simulink model "Noh_Nofusion"  (R2020b)
settings: Solver=FixedStepAuto  StartTime=0.0  StopTime=Inf  FixedStep=0.01  RelTol=1e-3
PostLoadFcn:
  | if any(exist('dsrtsu_mdlpostloadfcn', 'file') ~= 0), dsrtsu_mdlpostloadfcn('Execute', bdroot); end
InitFcn:
  | , if any(exist('rtifpga_mdlclblib', 'file') ~= 0), rtifpga_mdlclblib('Init', bdroot); end,
  | , if any(exist('dsmpb_private', 'file') ~= 0), dsmpb_private('dsmpb_mdlclblib', 'Init', bdroot); end,
undefined symbols (not defined in the file): ACC_TimeGap_DecSetSwt, ACC_TimeGap_IncSetSwt, AccelPedalPosn, AccelPedalPosnVldty, AccelPedlPosnDiagc, AccPedalOverride, ACU_ShiftInProgress, ADAS_Posn_CurLane, AESSwtReq, ALC_SwtReq, BrkPedalSts, CC_ACC_CANCEL_OFFSwt, CC_ACC_CRUISE_OFFSwt, CC_ACC_DecSetSpd_SetSwt, CC_ACC_IncSetSpd_ResuSwt, CC_ACCSwtErr, CharSpd_ms, CSA_NODE, CURRENT_GEAR, CurrentGearValid, DiscIntNeverNeededParam, DrvDoorSts, DrvSBR, DrvTrqReqOvld, ECMACCInterface, ECMRespACC, ELKSwtReq, EngLimpHomeSts, EngSpd, EngState, EngState_PHEV, EngTrqMaxActSpd, EngTrqMinAct, EPS_DrvInpTrqVal_HighReslolution, EPS_FailSts, EPS_LKATorqOvrlDlvd, EPS_LKATorqOvrlDlvdVld, EPS_LKATrqOvlDlvdSts, EPS_SteerMod, EPS_TrqSnsrSts, EQ4_APPINFO, EQ4_LA_ELEM, EQ4_LA_HDR, EQ4_LAP_ELEM, EQ4_LAP_HDR, EQ4_LH_ELEM, EQ4_LH_HDR, EQ4_LRE_ELEM, EQ4_LRE_HDR, ESS_PedSwtReq, ESS_VehSwtReq, FFogLmpSts_F_Pbox, FLWheelDriveDirection, FLWheelSpd, FrntWiprSwtSts, FrntWshrSwtSts, FRWheelDriveDirection, FRWheelSpd, HazardLmpSwtSts, HCU_AccelPedalPosn_Diag ... (+153)
libraries: simulink x132, dsmpblib x27
(part 14 of 14)

== matlab function Noh_Nofusion/TOS/Subsystem1/ACCOSM/HWA_Task100ms1/DycHistCalc ==
  data: TrajHistBufferBTrajEnd input boolean; ObjTrajNumber input uint8; ObjDycHist output single; TrajCurrentIndex input uint8; TrajHistBufferBValid input boolean; TrajHistBufferDxv input single; TrajHistBufferDyv input single; ObjValid input boolean; ObjqDycHist output single; dxC0 input; aP0 input; bP0 input; cP0 input; aP1 input; bP1 input; cP1 input
function [ObjDycHist,ObjqDycHist] = DycHistCalc(TrajHistBufferBTrajEnd,ObjTrajNumber,TrajCurrentIndex,...
    TrajHistBufferBValid,TrajHistBufferDxv,TrajHistBufferDyv,ObjValid,dxC0,aP0,bP0,cP0,aP1,bP1,cP1)

t_dxv = single(0);
t_dyv = single(0);
t_dxvK1 = single(0);
t_dyvK1 = single(0);
ObjDycHist = single(zeros(15,1));
ObjqDycHist = single(zeros(15,1));

for iObj=1:15
    t_TrajNumber = ObjTrajNumber(iObj);
    if t_TrajNumber<21
        t_End = false;
        t_Failed = false;
        t_TrajCurrentIndex = TrajCurrentIndex(t_TrajNumber);
        t_TrajEnd = TrajHistBufferBTrajEnd(t_TrajNumber,t_TrajCurrentIndex);
        if (ObjValid(iObj)==true)&&(t_TrajEnd==false)
            for k=1:24
                if t_End==false
                    if t_TrajCurrentIndex<k
                        t_Index = t_TrajCurrentIndex + uint8(25) - k;
                    else
                        t_Index = t_TrajCurrentIndex - k + uint8(1);
                    end
                    if t_Index==1
                        t_IndexK1 = uint8(24);
                    else
                        t_IndexK1 = t_Index - uint8(1);
                    end
                    t_ValidK1 = TrajHistBufferBValid(t_TrajNumber,t_IndexK1);
                    t_TrajEndK1 = TrajHistBufferBTrajEnd(t_TrajNumber,t_IndexK1);
                    t_dxv = TrajHistBufferDxv(t_TrajNumber,t_Index);
                    t_dxvK1 = TrajHistBufferDxv(t_TrajNumber,t_IndexK1);
                    t_dyv = TrajHistBufferDyv(t_TrajNumber,t_Index);
                    t_dyvK1 = TrajHistBufferDyv(t_TrajNumber,t_IndexK1);
                    
                    if (t_TrajEndK1==true)||(t_ValidK1==false)
                        t_End = true;
                        t_Failed = true;
                    end
                    if (t_dxv>=0)&&(t_dxvK1<=0)
                        t_End = true;
                    end
                end
            end
        end
        if (t_End==true)&&(t_Failed==false)
            if (t_dxv==t_dxvK1)
                t_dycHist = t_dyv;
            else
                t_dycHist = t_dyv - t_dxv*(t_dyvK1 - t_dyv)/(t_dxvK1 - t_dxv);
            end
            t_qDycHist = single(1);  
        else
            if (t_End==true)&&(t_Failed==true)&&(t_dxv>0)
                if t_dxv>(dxC0)
                    t_dycHist = t_dyv - (aP1*t_dxv*t_dxv + bP1*t_dxv + cP1); 
                else
                    t_dycHist = t_dyv - (aP0*t_dxv*t_dxv + bP0*t_dxv + cP0); 
                end
               t_qDycHist = max((single(80) - t_dxv)/single(80),single(0));
            else
                t_dycHist = single(0);
                t_qDycHist = single(0);
            end
        end
    else
        t_dycHist = single(0);
        t_qDycHist = single(0);
    end
    ObjDycHist(iObj) = t_dycHist;
    ObjqDycHist(iObj) = t_qDycHist;
end

== matlab function Noh_Nofusion/TOS/Subsystem1/ACCOSM/HWA_Task100ms1/LostTargetCalc ==
  data: ObjValid input boolean size=15; ReID output uint8 size=1; ObjDx input single size=15; ObjDy input single size=15; DeltaDx input single size=1; DeltaDy input single size=1; P0IDK1 input uint8 size=1; P0VxK1 input single size=1; P0DxK1 input single size=1; P0DyK1 input single size=1; P0RangeK1 input; P0ArGK1 input; P0DycK1 input single size=1; P0VycK1 input single size=1; P0CutIn_bK1 input boolean size=1; tTargetLostK1 input single size=1; ReRange output single size=1; ReArG output single size=1; ReDx output single size=1; ReDy output single size=1; ReVx output single size=1; ReCutIn_b output boolean size=1; ReDyc output single size=1; ReVyc output single size=1; TargetLost_b output boolean size=1; Covered_b output boolean size=1; tTargetLost output single size=1
function [ReID,ReRange,ReArG,ReDx,ReDy,ReVx,ReCutIn_b,ReDyc,ReVyc,TargetLost_b,Covered_b,tTargetLost]...
    = LostTargetCalc(ObjValid,ObjDx,ObjDy,DeltaDx,DeltaDy,...
    P0IDK1,P0VxK1,P0DxK1,P0DyK1,P0RangeK1,P0ArGK1,P0DycK1,P0VycK1,P0CutIn_bK1,tTargetLostK1)
 
ReID = P0IDK1;
ReRange = single(255);
ReArG = single(0);
ReDx = single(255);
ReDy = single(0);
ReVx = single(0);
ReDyc = single(0);
ReVyc = single(0);
ReCutIn_b = false;
TargetLost_b = false;
tTargetLost = single(0);
Covered_b = false;
 
if (P0IDK1>0)&&(P0IDK1<100)    % k1 Exist Target
    if ObjValid(P0IDK1)==false
        ExistNearObj = false;
        P0DxPred = P0DxK1 + 0.1*P0VxK1;
        P0DyPred = P0DyK1;
        P0RangePred = P0RangeK1 + 0.1*P0VxK1; 
        for i=1:15
            if (ObjValid(i)==true)&&(ObjDx(i)<P0DxPred)
                Covered_b = CoveredCalc(P0DxPred,P0DyPred,ObjDx(i),ObjDy(i),single(2.1),single(-0.1));
                if Covered_b==true
                   break; 
                end
            end
            if (ObjValid(i)==1)&&(abs(ObjDx(i)-P0DxPred)<DeltaDx)&&(abs(ObjDy(i)-P0DyPred)<DeltaDy)
               ExistNearObj = true;
               ReID = uint8(i);
               ReDx = ObjDx(i);
            end
        end
        if (ExistNearObj==false)&&(Covered_b==false)
            TargetLost_b = true;
            tTargetLost = single(0.1);
            ReID = uint8(255);
            ReRange = P0RangePred;
            ReArG = P0ArGK1;
            ReDx = P0DxPred;
            ReDy = P0DyPred;
            ReVx = P0VxK1;
            ReCutIn_b = P0CutIn_bK1;
            ReVyc = P0VycK1;
            ReDyc = P0DycK1 + 0.1*P0VycK1;
        end
    end
else
    if P0IDK1>100   %  k1 Exist Target Re
        ExistNearObj = false;
        P0DxPred = P0DxK1 + 0.1*P0VxK1;
        P0DyPred = P0DyK1;
        P0RangePred = P0RangeK1 + 0.1*P0VxK1; 

        for i=1:15
            if (ObjValid(i)==1)&&(abs(ObjDx(i)-P0DxPred)<DeltaDx)&&(abs(ObjDy(i)-P0DyPred)<DeltaDy)
                ExistNearObj = true;
                ReID = uint8(i);
                ReDx = ObjDx(i);
                TargetLost_b = false;
                tTargetLost = single(0);
            end
        end
        if ExistNearObj==false
            TargetLost_b = true;
            tTargetLost = tTargetLostK1 + single(0.1);
            ReID = uint8(255);
            ReRange = P0RangePred;
            ReArG = P0ArGK1;
            ReDx = P0DxPred;
            ReDy = P0DyPred;
            ReVx = P0VxK1;
            ReCutIn_b = P0CutIn_bK1;
            ReVyc = P0VycK1;
            ReDyc = P0DycK1 + 0.1*P0VycK1;
        end
    end
end
end
 
function t_Covered_b = CoveredCalc(DxPred,DyPred,Dx,Dy,IFVDx,IFVDy)
y = (IFVDy - DyPred)*(Dx - DxPred)/(IFVDx - DxPred) + DyPred ;
Delta = single(0.8) + (Dx - IFVDx)/(DxPred - IFVDx);
if abs(Dy - y)<=Delta
    t_Covered_b = true;
else
    t_Covered_b = false;
end
end

== matlab function Noh_Nofusion/TOS/Subsystem1/ACCOSM/HWA_Task100ms1/Lpb ==
  data: vRef input single size=1; alpSumSlideCurveness input single size=1; ObjValid input boolean size=15; ObjDyc input single size=15; ObjLpb output single size=15; ObjDycHist input single size=15; ObjqDycHist input single size=15; ObjLpbL output single size=15; ObjLpbR output single size=15; ObjVyc input single size=15; ObjYawAngle input single size=15; ObjDylaneEdgeRight input; ObjDyEdgeWidthRight input; ObjDylaneEdgeLeft input; ObjDyEdgeWidthLeft input
function [ObjLpb,ObjLpbL,ObjLpbR] = LpbCalc(vRef,alpSumSlideCurveness,...
    ObjValid,ObjDyc,ObjDycHist,ObjqDycHist,ObjVyc,ObjYawAngle,...
    ObjDylaneEdgeRight,ObjDyEdgeWidthRight,ObjDylaneEdgeLeft,ObjDyEdgeWidthLeft)

 [ObjLpb,ObjLpbL,ObjLpbR] = LpbCalc(vRef,alpSumSlideCurveness,...
    ObjValid,ObjDyc,ObjDycHist,ObjqDycHist,ObjVyc,ObjYawAngle,...
    ObjDylaneEdgeRight,ObjDyEdgeWidthRight,ObjDylaneEdgeLeft,ObjDyEdgeWidthLeft);
end

== matlab function Noh_Nofusion/TOS/Subsystem1/ACCOSM/HWA_Task100ms1/OTL1/MATLAB Function ==
  data: t input single; Valid output boolean; CutIn_b input boolean; ValidK1 input boolean
function Valid = fcn(t,CutIn_b,ValidK1)

if t<0.1
    Valid = false;
else
    if CutIn_b==false
       Valid = true; 
    else
       Valid = ValidK1;
    end
end

== matlab function Noh_Nofusion/TOS/Subsystem1/ACCOSM/HWA_Task100ms1/OTL1/P0TrajHistCalc01 ==
  data: P0Dyc output; vRef input; tCycle input single; tSameHandle input single; CutIn input; P0Dx input single; P0Dy input single; P0TrajHistNum output uint8; EgoDDeltaX input single; EgoDDeltaY input single; EgoCosOfPsi input single; EgoSinOfPsi input single; TarLineValid input; TarLineA2 input; TarLineA1 input; TarLineA0 input; P0TrajHistDxv output single; P0TrajHistDyv output single; P0TrajHistNumK1 input uint8; P0TrajHistDxvK1 input single; P0TrajHistDyvK1 input single
function [P0Dyc,P0TrajHistNum,P0TrajHistDxv,P0TrajHistDyv]...
    = fcn(vRef, tCycle,tSameHandle,CutIn, P0Dx,P0Dy,EgoDDeltaX,EgoDDeltaY,EgoCosOfPsi,EgoSinOfPsi,...
    TarLineValid,TarLineA2,TarLineA1,TarLineA0,...
    P0TrajHistNumK1,P0TrajHistDxvK1,P0TrajHistDyvK1)
%#codegen
P0TrajHistNum = P0TrajHistNumK1;
P0TrajHistDxv = P0TrajHistDxvK1;
P0TrajHistDyv = P0TrajHistDyvK1;

if TarLineValid
    temp1 = TarLineA2*P0Dx*P0Dx + TarLineA1*P0Dx + TarLineA0;
    P0Dyc = P0Dy - temp1;
else
    P0Dyc = single(255);
end
                
if tSameHandle==0
    P0TrajHistNum = uint8(0);
    P0TrajHistDxv = single(zeros(24,1));
    P0TrajHistDyv = single(zeros(24,1));
else
    if tSameHandle==tCycle
        if (CutIn&&abs(P0Dyc)>0.5) || (abs(P0Dyc)>0.8)||(vRef>8)
            P0TrajHistDxv(1) = P0Dx;
            P0TrajHistDyv(1) = P0Dy;
            P0TrajHistNum = uint8(1);
        else
            P0TrajHistDxv(1) = P0Dx;
            P0TrajHistDyv(1) = P0Dy;
            P0TrajHistNum = uint8(1);
            
            if TarLineValid
                P0TrajHistDxv(2) = 0.6*P0Dx;
                temp2 = 0.36*TarLineA2*P0Dx*P0Dx + 0.6*TarLineA1*P0Dx + TarLineA0;
                P0TrajHistDyv(2) = P0Dyc + temp2;
                
                P0TrajHistDxv(3) = 0.3*P0Dx;
                temp3 = 0.09*TarLineA2*P0Dx*P0Dx + 0.3*TarLineA1*P0Dx + TarLineA0;
                P0TrajHistDyv(3) = P0Dyc + temp3;
                
                P0TrajHistDxv(4) = single(-1);
                temp4 = TarLineA2 - TarLineA1 + TarLineA0;
                P0TrajHistDyv(4) = P0Dyc + temp4;
                
                P0TrajHistNum = uint8(4);
            end
        end
    else
        Temp1 = P0TrajHistDxv(1) - EgoDDeltaX - P0Dx;
        Temp2 = P0TrajHistDyv(1) - EgoDDeltaY - P0Dy;
        dDeltaS = Temp1*Temp1 + Temp2*Temp2;
        
        t_d = interpolate(single(8),single(0.5),single(22),single(2.5),single(P0TrajHistNum));
        t_d = t_d*t_d;
        t_AddPosition = (dDeltaS>t_d);
        
        for iBuf=1:P0TrajHistNum
            dX = P0TrajHistDxv(iBuf)-EgoDDeltaX;
            dY = P0TrajHistDyv(iBuf)-EgoDDeltaY;
            P0TrajHistDxv(iBuf) = dX*EgoCosOfPsi + dY*EgoSinOfPsi;
            P0TrajHistDyv(iBuf) = -dX*EgoSinOfPsi + dY*EgoCosOfPsi;
            if (P0TrajHistDxv(iBuf)<-5)||(abs(P0TrajHistDyv(iBuf))>50)
                P0TrajHistNum = max(P0TrajHistNum - uint8(1),uint8(0));
            end
        end
        
        if t_AddPosition==true
            
            P0TrajHistNum = min(P0TrajHistNum + uint8(1),uint8(24));
            for iBuf= P0TrajHistNum:(-1):2
                P0TrajHistDxv(iBuf) = P0TrajHistDxv(iBuf-uint8(1));
                P0TrajHistDyv(iBuf) = P0TrajHistDyv(iBuf-uint8(1));
            end
            P0TrajHistDxv(1) = P0Dx;
            P0TrajHistDyv(1) = P0Dy;
        end
    end
end
end

function out = interpolate(x1,z1,x2,z2,Raw)
if Raw<=x1
    out = z1;
else
    if Raw>=x2
        out = z2;
    else
        out = z1 + (Raw-x1)*(z2-z1)/(x2-x1);
    end
end
end

== matlab function Noh_Nofusion/Subsystem4/LALine ==
  data: LA_Count input; L1Conf output uint8 size=1; L1C0 output single size=1; L1C1 output single size=1; L1C2 output single size=1; L1C3 output single size=1; L1DxMin output single size=1; L1DxMax output single size=1; L1A0 input single size=1; L1A1 input single size=1; L1A2 input single size=1; L1A3 input single size=1; L1RaMin input single size=1; L1RaMax input single size=1; L1Avail input uint8 size=1; L1LineType input uint8 size=1; L1DLType input uint8 size=1; L1SideType input uint8 size=1; L1Wid input single size=1; L1Confidence input; L2A0 input single size=1; L2A1 input single size=1; L2A2 input single size=1; L2A3 input single size=1; L2RaMin input single size=1; L2RaMax input single size=1; L2Avail input uint8 size=1; L2LineType input uint8 size=1; L2DLType input uint8 size=1; L2SideType input uint8 size=1; L2Wid input single size=1; L2Confidence input; L3A0 input single size=1; L3A1 input single size=1; L3A2 input single size=1; L3A3 input single size=1; L3RaMin input single size=1; L3RaMax input single size=1; L3Avail input uint8 size=1; L3LineType input uint8 size=1; L3DLType input uint8 size=1; L3SideType input uint8 size=1; L3Wid input single size=1; L3Confidence input; L4A0 input single size=1; L4A1 input single size=1; L4A2 input single size=1; L4A3 input single size=1; L4RaMin input single size=1; L4RaMax input single size=1; L4Avail input uint8 size=1; L4LineType input uint8 size=1; L4DLType input uint8 size=1; L4SideType input uint8 size=1; L4Wid input single size=1; L1Type output uint8 size=1; L1DLM output uint8 size=1; L1Width output single size=1; L1Reliable output; L2Conf output uint8 size=1; L2C0 output single size=1; L2C1 output single size=1; L2C2 output single size=1; L2C3 output single size=1; L2DxMin output single size=1; L2DxMax output single size=1; L2Type output uint8 size=1; L2DLM output uint8 size=1; L2Width output single size=1; L2Reliable output; L3Conf output uint8 size=1; L3C0 output single size=1; L3C1 output single size=1; L3C2 output single size=1; L3C3 output single size=1; L3DxMin output single size=1; L3DxMax output single size=1; L3Type output uint8 size=1; L3DLM output uint8 size=1; L3Width output single size=1; L3Reliable output; L4Conf output uint8 size=1; L4C0 output single size=1; L4C1 output single size=1; L4C2 output single size=1; L4C3 output single size=1; L4DxMin output single size=1; L4DxMax output single size=1; L4Type output uint8 size=1; L4DLM output uint8 size=1; L4Width output single size=1; L4Confidence input; L4Reliable output
function [L1Conf,L1C0,L1C1,L1C2,L1C3,L1DxMin,L1DxMax,L1Type,L1DLM,L1Width,L1Reliable,...
    L2Conf,L2C0,L2C1,L2C2,L2C3,L2DxMin,L2DxMax,L2Type,L2DLM,L2Width,L2Reliable,...
    L3Conf,L3C0,L3C1,L3C2,L3C3,L3DxMin,L3DxMax,L3Type,L3DLM,L3Width,L3Reliable,...
    L4Conf,L4C0,L4C1,L4C2,L4C3,L4DxMin,L4DxMax,L4Type,L4DLM,L4Width,L4Reliable]...
    = LA(LA_Count,L1A0,L1A1,L1A2,L1A3,L1RaMin,L1RaMax,L1Avail,L1LineType,L1DLType,L1SideType,L1Wid,L1Confidence,...
    L2A0,L2A1,L2A2,L2A3,L2RaMin,L2RaMax,L2Avail,L2LineType,L2DLType,L2SideType,L2Wid,L2Confidence,...
    L3A0,L3A1,L3A2,L3A3,L3RaMin,L3RaMax,L3Avail,L3LineType,L3DLType,L3SideType,L3Wid,L3Confidence,...
    L4A0,L4A1,L4A2,L4A3,L4RaMin,L4RaMax,L4Avail,L4LineType,L4DLType,L4SideType,L4Wid,L4Confidence)

L1Conf = uint8(0);
L1C0 = single(0);
L1C1 = single(0);
L1C2 = single(0);
L1C3 = single(0);
L1DxMin = single(0);
L1DxMax = single(0);
L1Type = uint8(0);
L1DLM = uint8(0);
L1Width = single(0);
L1Reliable = single(0);

L2Conf = uint8(0);
L2C0 = single(0);
L2C1 = single(0);
L2C2 = single(0);
L2C3 = single(0);
L2DxMin = single(0);
L2DxMax = single(0);
L2Type = uint8(0);
L2DLM = uint8(0);
L2Width = single(0);
L2Reliable = single(0);

L3Conf = uint8(0);
L3C0 = single(0);
L3C1 = single(0);
L3C2 = single(0);
L3C3 = single(0);
L3DxMin = single(0);
L3DxMax = single(0);
L3Type = uint8(0);
L3DLM = uint8(0);
L3Width = single(0);
L3Reliable = single(0);

L4Conf = uint8(0);
L4C0 = single(0);
L4C1 = single(0);
L4C2 = single(0);
L4C3 = single(0);
L4DxMin = single(0);
L4DxMax = single(0);
L4Type = uint8(0);
L4DLM = uint8(0);
L4Width = single(0);
L4Reliable = single(0);
%%  临车道车道线预处理
if LA_Count >= 1                                     %临车道车道线数量
    if L1SideType==1                                 %左左车道线
        L1Conf = L1Avail;
        L1C0 = L1A0;
        L1C1 = L1A1;
        L1C2 = L1A2;
        L1C3 = L1A3;
        L1DxMin = L1RaMin;
        L1DxMax = L1RaMax;
        L1Type = L1LineType;
        L1DLM = L1DLType;
        L1Width = L1Wid;
        L1Reliable = L1Confidence;
    elseif L1SideType==2                             %左车道右侧车道线
        L2Conf = L1Avail;
        L2C0 = L1A0;
        L2C1 = L1A1;
        L2C2 = L1A2;
        L2C3 = L1A3;
        L2DxMin = L1RaMin;
        L2DxMax = L1RaMax;
        L2Type = L1LineType;
        L2DLM = L1DLType;
        L2Width = L1Wid;
        L2Reliable = L1Confidence;
    elseif L1SideType==3                             %右车道左侧车道线
        L3Conf = L1Avail;
        L3C0 = L1A0;
        L3C1 = L1A1;
        L3C2 = L1A2;
        L3C3 = L1A3;
        L3DxMin = L1RaMin;
        L3DxMax = L1RaMax;
        L3Type = L1LineType;
        L3DLM = L1DLType;
        L3Width = L1Wid;
        L3Reliable = L1Confidence;
    elseif L1SideType==4                             %右右车道线
        L4Conf = L1Avail;
        L4C0 = L1A0;
        L4C1 = L1A1;
        L4C2 = L1A2;
        L4C3 = L1A3;
        L4DxMin = L1RaMin;
        L4DxMax = L1RaMax;
        L4Type = L1LineType;
        L4DLM = L1DLType;
        L4Width = L1Wid;
        L4Reliable = L1Confidence;
    end
    if LA_Count >= 2
        if L2SideType==1
            L1Conf = L2Avail;
            L1C0 = L2A0;
            L1C1 = L2A1;
            L1C2 = L2A2;
            L1C3 = L2A3;
            L1DxMin = L2RaMin;
            L1DxMax = L2RaMax;
            L1Type = L2LineType;
            L1DLM = L2DLType;
            L1Width = L2Wid;
            L1Reliable = L2Confidence;
        elseif L2SideType==2
            L2Conf = L2Avail;
            L2C0 = L2A0;
            L2C1 = L2A1;
            L2C2 = L2A2;
            L2C3 = L2A3;
            L2DxMin = L2RaMin;
            L2DxMax = L2RaMax;
            L2Type = L2LineType;
            L2DLM = L2DLType;
            L2Width = L2Wid;
            L2Reliable = L2Confidence;
        elseif L2SideType==3
            L3Conf = L2Avail;
            L3C0 = L2A0;
            L3C1 = L2A1;
            L3C2 = L2A2;
            L3C3 = L2A3;
            L3DxMin = L2RaMin;
            L3DxMax = L2RaMax;
            L3Type = L2LineType;
            L3DLM = L2DLType;
            L3Width = L2Wid;
            L3Reliable = L2Confidence;
        elseif L2SideType==4
            L4Conf = L2Avail;
            L4C0 = L2A0;
            L4C1 = L2A1;
            L4C2 = L2A2;
            L4C3 = L2A3;
            L4DxMin = L2RaMin;
            L4DxMax = L2RaMax;
            L4Type = L2LineType;
            L4DLM = L2DLType;
            L4Width = L2Wid;
            L4Reliable = L2Confidence;
        end
        if LA_Count >= 3
            if L3SideType==1
                L1Conf = L3Avail;
                L1C0 = L3A0;
                L1C1 = L3A1;
                L1C2 = L3A2;
                L1C3 = L3A3;
                L1DxMin = L3RaMin;
                L1DxMax = L3RaMax;
                L1Type = L3LineType;
                L1DLM = L3DLType;
                L1Width = L3Wid;
                L1Reliable = L3Confidence;
            elseif L3SideType==2
                L2Conf = L3Avail;
                L2C0 = L3A0;
                L2C1 = L3A1;
                L2C2 = L3A2;
                L2C3 = L3A3;
                L2DxMin = L3RaMin;
                L2DxMax = L3RaMax;
                L2Type = L3LineType;
                L2DLM = L3DLType;
                L2Width = L3Wid;
                L2Reliable = L3Confidence;
            elseif L3SideType==3
                L3Conf = L3Avail;
                L3C0 = L3A0;
                L3C1 = L3A1;
                L3C2 = L3A2;
                L3C3 = L3A3;
                L3DxMin = L3RaMin;
                L3DxMax = L3RaMax;
                L3Type = L3LineType;
                L3DLM = L3DLType;
                L3Width = L3Wid;
                L3Reliable = L3Confidence;
            elseif L3SideType==4
                L4Conf = L3Avail;
                L4C0 = L3A0;
                L4C1 = L3A1;
                L4C2 = L3A2;
                L4C3 = L3A3;
                L4DxMin = L3RaMin;
                L4DxMax = L3RaMax;
                L4Type = L3LineType;
                L4DLM = L3DLType;
                L4Width = L3Wid;
                L4Reliable = L3Confidence;
            end
            if LA_Count >= 4
                if L4SideType==1
                    L1Conf = L4Avail;
                    L1C0 = L4A0;
                    L1C1 = L4A1;
                    L1C2 = L4A2;
                    L1C3 = L4A3;
                    L1DxMin = L4RaMin;
                    L1DxMax = L4RaMax;
                    L1Type = L4LineType;
                    L1DLM = L4DLType;
                    L1Width = L4Wid;
                    L1Reliable = L4Confidence;
                elseif L4SideType==2
                    L2Conf = L4Avail;
                    L2C0 = L4A0;
                    L2C1 = L4A1;
                    L2C2 = L4A2;
                    L2C3 = L4A3;
                    L2DxMin = L4RaMin;
                    L2DxMax = L4RaMax;
                    L2Type = L4LineType;
                    L2DLM = L4DLType;
                    L2Width = L4Wid;
                    L2Reliable = L4Confidence;
                elseif L4SideType==3
                    L3Conf = L4Avail;
                    L3C0 = L4A0;
                    L3C1 = L4A1;
                    L3C2 = L4A2;
                    L3C3 = L4A3;
                    L3DxMin = L4RaMin;
                    L3DxMax = L4RaMax;
                    L3Type = L4LineType;
                    L3DLM = L4DLType;
                    L3Width = L4Wid;
                    L3Reliable = L4Confidence;
                elseif L4SideType==4
                    L4Conf = L4Avail;
                    L4C0 = L4A0;
                    L4C1 = L4A1;
                    L4C2 = L4A2;
                    L4C3 = L4A3;
                    L4DxMin = L4RaMin;
                    L4DxMax = L4RaMax;
                    L4Type = L4LineType;
                    L4DLM = L4DLType;
                    L4Width = L4Wid;
                    L4Reliable = L4Confidence;
                end
            end
        end
    end
end

== matlab function Noh_Nofusion/TOS/Subsystem1/ACCOSM/HWA_Task100ms1/OTL1/P0TrajHistCalc1 ==
  data: P0TrajHistNum output uint8; P0TrajHistNum1 input uint8; P0TrajHistDxv1 input single; P0TrajHistDxv output single; P0TrajHistDyv1 input single; P0TrajHistDyv output single; LineValid output boolean; a output single; b output single; c output single; d output single; dxMin output single; dxMax output single
function [P0TrajHistNum,P0TrajHistDxv,P0TrajHistDyv,LineValid,a,b,c,d,dxMin,dxMax] = P0TrajHistMixCalc(...
    P0TrajHistNum1,P0TrajHistDxv1,P0TrajHistDyv1)

P0TrajHistDxv = single(zeros(48,1));
P0TrajHistDyv = single(zeros(48,1));
P0TrajHistNum = uint8(0);

if (P0TrajHistNum1>0)
    P0TrajHistDxv(1:P0TrajHistNum1) = P0TrajHistDxv1(1:P0TrajHistNum1);
    P0TrajHistDyv(1:P0TrajHistNum1) = P0TrajHistDyv1(1:P0TrajHistNum1);
    P0TrajHistNum = P0TrajHistNum1;
end

if P0TrajHistNum>=4
    dxMin = P0TrajHistDxv(P0TrajHistNum);
    dxMax = P0TrajHistDxv(1) + 6;
%     q2 = max(ceil(P0TrajHistNum/2),2);
%     q3 = max(ceil(P0TrajHistNum*3/4),3);
%     q4 = P0TrajHistNum;
%     MaX = [P0TrajHistDxv(1);P0TrajHistDxv(q2);P0TrajHistDxv(q3);P0TrajHistDxv(q4)];
%     MaY = [P0TrajHistDyv(1);P0TrajHistDyv(q2);P0TrajHistDyv(q3);P0TrajHistDyv(q4)];
%     [~,b,c,d] = pl(MaX,MaY);
    P = polyfit(P0TrajHistDxv(1:P0TrajHistNum),P0TrajHistDyv(1:P0TrajHistNum),2);
    b = P(1);
    c = P(2);
    d = P(3);

    a = single(0);
   LineValid = true;
   if dxMin>0.5
      LineValid = false; 
   end
else
   dxMin = single(0); 
   dxMax = single(0); 
   a = single(0);
   b = single(0);
   c = single(0);
   d = single(0);
   LineValid = false;
end

== matlab function Noh_Nofusion/TOS/Subsystem1/ACCOSM/HWA_Task100ms1/Plaus ==
  data: dxMaxFollow input single size=1; ObjValid input boolean size=15; ObjDx input single size=15; ObjVx input single size=15; ObjPlaus output single size=15; ObjOnLeft input single size=15; ObjPlausLeft output single size=15; ObjPlausRight output single size=15; ObjOnRight input single size=15; ObjDycHist input single size=15; ObjqDycHist input single size=15; ObjLpb input single size=15; ObjLpbLeft input single size=15; ObjLpbRight input single size=15; ObjPlausK1 input single size=15; ObjPlausLeftK1 input single size=15; ObjPlausRightK1 input single size=15
function [ObjPlaus,ObjPlausLeft,ObjPlausRight] = ...
    PlausCalc(dxMaxFollow,ObjValid,ObjDx,ObjVx,ObjOnLeft,ObjOnRight,ObjDycHist,ObjqDycHist,...
    ObjLpb,ObjLpbLeft,ObjLpbRight,ObjPlausK1,ObjPlausLeftK1,ObjPlausRightK1)

[ObjPlaus,ObjPlausLeft,ObjPlausRight] = ...
    PlausCalc(dxMaxFollow,ObjValid,ObjDx,ObjVx,ObjOnLeft,ObjOnRight,ObjDycHist,ObjqDycHist,...
    ObjLpb,ObjLpbLeft,ObjLpbRight,ObjPlausK1,ObjPlausLeftK1,ObjPlausRightK1);
end

== matlab function Noh_Nofusion/TOS/Subsystem1/ACCOSM/HWA_Task100ms1/Spw ==
  data: AlpSumSlideCurveness input single size=1; kapCourseErr input single size=1; ObjSpw output single size=15; ObjValid input boolean size=15; DycASI input single size=15; ObjDx input single size=15; ObjSpwLeft output single size=15; ObjSpwRight output single size=15; ObjOnLeft output; ObjOnRight output; ObjDyc input; ObjDycHist input; ObjqDycHist input; ObjDycASI output; ObjDyKapErr output
function [ObjSpw,ObjSpwLeft,ObjSpwRight,ObjOnLeft,ObjOnRight,ObjDycASI,ObjDyKapErr] = ...
    CalcSpw(AlpSumSlideCurveness,kapCourseErr,ObjValid,DycASI,ObjDx,ObjDyc,ObjDycHist,ObjqDycHist)
 
ObjSpw = single(zeros(15,1));
ObjSpwLeft = single(zeros(15,1));
ObjSpwRight = single(zeros(15,1));
ObjOnLeft = single(zeros(15,1));
ObjOnRight = single(zeros(15,1));
ObjDycASI = single(zeros(15,1));
ObjDyKapErr = single(zeros(15,1));
 
for i=1:15
    if ObjValid(i)
        t_dycASI = DycASI(i);
        t_kapErrMin = single(0.0002);
        t_kapErrCurvenessMax = single(0.0018);
        
        temp1 = min(AlpSumSlideCurveness,single(1));
        t_kapErrCurveness = t_kapErrCurvenessMax*temp1;
        t_kapErr = max(t_kapErrMin,max(kapCourseErr,t_kapErrCurveness));
        temp1 = min(ObjDx(i),single(80));
        t_DyKapErr = t_kapErr*temp1*temp1/2;
        ObjDyKapErr(i) = t_DyKapErr;
        
        %         t_dyHalfLane = 1.5;
        %         t_dy3halfLane = 5.25;
        
        if abs(t_dycASI)>=4.5
            t_spw = single(0);
            t_spwNeighbour = single(0);
        elseif abs(t_dycASI)>=3
            t_spw = single(0);
            t_dycToLane = abs(t_dycASI) - single(3);
            t_spwNeighbour = CalcSPW(t_dycToLane,single(3),t_DyKapErr);
        elseif abs(t_dycASI)>=1.5
            t_spw = single(0);
            t_spwNeighbour = CalcSPW(single(0),single(3),t_DyKapErr);
        else
            t_spwNeighbour = single(0);
            t_spw = CalcSPW(single(0),single(3),t_DyKapErr);
        end
        if t_dycASI>=0
            t_spwRight = single(0);
            t_spwLeft = t_spwNeighbour;
        else
            t_spwLeft = single(0);
            t_spwRight = t_spwNeighbour;
        end
        ObjSpw(i) = t_spw;
        ObjSpwLeft(i) = t_spwLeft;
        ObjSpwRight(i) = t_spwRight;
        % -------------------------------------------------------------------------
        
        temp1 = 0.5*ObjqDycHist(i);
        t_dycASI = ObjDyc(i)*(1-temp1) + ObjDycHist(i)*temp1;
        temp2 = single(1.5) + t_DyKapErr;
        temp3 = single(3) + t_DyKapErr;
        ObjDycASI(i) = t_dycASI;
        
        if t_dycASI>=0
            temp1 = max(single(1.5),min(temp3,t_dycASI)) - single(1.5);
            ObjOnLeft(i) = min(single(1),temp1/temp2);
        else
            temp1 = max(min(single(-1.5),t_dycASI),-temp3);
            temp1 = -temp1 - single(1.5);
            ObjOnRight(i) = min(single(1),temp1/temp2);
        end
    end
end
end
 
function t_spw = CalcSPW(absDyc,dyLaneWidth,dyKapErr)
temp3 = dyLaneWidth/2;
temp1 = temp3 - dyKapErr;
temp2 = temp3 + dyKapErr;
temp2 = min(temp2,dyLaneWidth);
 
if absDyc<=temp1
    t_spw = single(1);
elseif absDyc>=temp2
    t_spw = single(0);
else
    temp3 = temp2 - absDyc;
    temp4 = 2*dyKapErr;
    t_spw = temp3/temp4;
end
end

== matlab function Noh_Nofusion/TOS/Subsystem1/ACCOSM/HWA_Task100ms1/Std ==
  data: u input; y output
function y = fcn(u)

y = std(u);

== matlab function Noh_Nofusion/TOS/Subsystem1/ACCOSM/HWA_Task100ms1/TargetBrake ==
  data: ID input uint8; VxG input; VyG input; TargetBrake_b output boolean; TargetVxG output; BrakeLightIndic input uint8 size=15; TargetVyG output
function [TargetBrake_b,TargetVxG,TargetVyG] = fcn(ID,VxG,VyG,BrakeLightIndic)
%#codegen
TargetBrake_b = false;
TargetVxG = single(0);
TargetVyG = single(0);

if (ID>0)&&(ID<100)
    if BrakeLightIndic(ID)==2
        TargetBrake_b = true;
    end
    TargetVxG = VxG(ID);
    TargetVyG = VyG(ID);
end

== matlab function Noh_Nofusion/TOS/Subsystem1/ACCOSM/HWA_Task100ms1/TargetSelect ==
  data: ACCmode input uint8 size=1; P0ID output uint8 size=1; vRef input single size=1; Valid input boolean size=15; Range input single size=15; Vr input single size=15; Dx input single size=15; Dy input single size=15; ArG input single size=15; Dyc input single size=15; Vyc input single size=15; Cnt input; plaus input single size=15; wCutIn input single size=15; spw input single size=15; spwLeft input single size=15; spwRight input single size=15; ReID input uint8 size=1; ReRange input single size=1; ReArG input single size=1; ReDx input single size=1; ReDy input single size=1; ReVx input single size=1; ReCutIn_b input boolean size=1; ReDyc input single size=1; ReVyc input single size=1; TargetLost_b input; tTargetLost input single size=1; dyLaneWidth input single size=1; Classfication input uint8 size=15; MoveSts input uint8 size=15; TarLimDx input single size=1; TarLimS0Dx input; TargetExistK1 input boolean size=1; P2ID output uint8 size=1; P3ID output uint8 size=1; P0Range output single size=1; P2Range output single size=1; P3Range output single size=1; P0Vr output single size=1; P2Vr output single size=1; P3Vr output single size=1; P0ArG output single size=1; P2ArG output single size=1; P3ArG output single size=1; P0Dx output single size=1; P2Dx output single size=1; P3Dx output single size=1; P0Dy output single size=1; P2Dy output single size=1; P3Dy output single size=1; TargetCutIn_b output boolean size=1; P0Dyc output single size=1; P0Vyc output single size=1; TargetExist output boolean size=1; TargetReplacedCntK1 input uint8; TargetReplacedCnt output uint8
function [P0ID,P2ID,P3ID,P0Range,P2Range,P3Range,P0Vr,P2Vr,P3Vr,P0ArG,P2ArG,P3ArG,...
    P0Dx,P2Dx,P3Dx,P0Dy,P2Dy,P3Dy,TargetCutIn_b,P0Dyc,P0Vyc,TargetExist,TargetReplacedCnt] = ...
    ATS(ACCmode,vRef,Valid,Range,Vr,Dx,Dy,ArG,Dyc,Vyc,Cnt,plaus,wCutIn,spw,spwLeft,spwRight,...
    ReID,ReRange,ReArG,ReDx,ReDy,ReVx,ReCutIn_b,ReDyc,ReVyc,TargetLost_b,tTargetLost,dyLaneWidth,...
    Classfication,MoveSts,TarLimDx,TarLimS0Dx,TargetExistK1,TargetReplacedCntK1)

% #codegen
% ACCMode
% 0x00:OFF mode
% 0x01:Passive mode(Reject)
% 0x02:Passive mode(Stand-by)
% 0x03:Active-Control mode
% 0x04:Brake-only mode
% 0x05:Override
% 0x06:Standstill
% 0x07:Failure mode
% 0x08~0x1F:Reserved

P0ID = uint8(0);
P2ID = uint8(0);
P3ID = uint8(0);
P0Range = single(255);
P2Range = single(255);
P3Range = single(255);
P0Vr = single(0);
P2Vr = single(0);
P3Vr = single(0);
P0ArG = single(0);
P2ArG = single(0);
P3ArG = single(0);
P0Dx = single(255);
P2Dx = single(255);
P3Dx = single(255);
P0Dy = single(0);
P2Dy = single(0);
P3Dy = single(0);
TargetExist = false;
TargetCutIn_b = false;
P0Dyc = single(0);
P0Vyc = single(0);

DycOffset = interpolate(single(50),single(0.35),single(80),single(0.6),ReDx);

if TargetLost_b
   TargetReplacedCnt = uint8(0);
else
   TargetReplacedCnt = min(uint8(255),TargetReplacedCntK1 + uint8(1));
end

if (ACCmode==1)||(ACCmode==2)||(ACCmode==3)||(ACCmode==4)||(ACCmode==5)||(ACCmode==6)||(ACCmode==9)
    if TargetExistK1==false   % first select target
        for i=1:15
            if (Valid(i)==1)&&(Cnt(i)>=3)&&...
                    (((vRef<=15.83)&&((MoveSts(i)==1)||(MoveSts(i)==2)||(MoveSts(i)==3)))||...
                    ((vRef>15.83)&&((MoveSts(i)==2)||(MoveSts(i)==3))))
                if (Classfication(i)==1)||(Classfication(i)==2)||(Classfication(i)==3)||(Classfication(i)==9)
                    if ((Range(i)<=TarLimS0Dx)&&(MoveSts(i)==1))||((Range(i)<=TarLimDx)&&((MoveSts(i)==2)||(MoveSts(i)==3)))
                        if (plaus(i)>=0.4)||((wCutIn(i)>0.7)&&(spw(i)>=0.8))||((spw(i)>0.95)&&(Range(i)<1.5*vRef))         % Need Check!
                            if Range(i)<P0Range
                                P0ID = uint8(i);
                                P0Range = Range(i);
                            end
                        else
                            if spwLeft(i)>0.2
                                if Range(i)<P2Range
                                    P2ID = uint8(i);
                                    P2Range = Range(i);
                                end
                            end
                            if spwRight(i)>0.2
                                if Range(i)<P3Range
                                    P3ID = uint8(i);
                                    P3Range = Range(i);
                                end
                            end
                        end
                    end
                end
            end
        end
    else
        k = ReID;
        if k<100        % No Target Lost!!!
            if (Valid(k)==0)
                for i=1:15
                    if (Valid(i)==1)&&...
                            (((vRef<=15.83)&&((MoveSts(i)==1)||(MoveSts(i)==2)||(MoveSts(i)==3)))||...
                            ((vRef>15.83)&&((MoveSts(i)==2)||(MoveSts(i)==3))))
                        if (Classfication(i)==1)||(Classfication(i)==2)||(Classfication(i)==3)||(Classfication(i)==9)
                            if ((Range(i)<=TarLimS0Dx)&&(MoveSts(i)==1))||((Range(i)<=TarLimDx)&&((MoveSts(i)==2)||(MoveSts(i)==3)))
                                if (plaus(i)>=0.4)||((wCutIn(i)>0.7)&&(spw(i)>=0.8))||((spw(i)>0.95)&&(Range(i)<1.5*vRef))
                                    if Range(i)<P0Range
                                        P0ID = uint8(i);
                                        P0Range = Range(i);
                                    end
                                else
                                    if spwLeft(i)>0.2
                                        if Range(i)<P2Range
                                            P2ID = uint8(i);
                                            P2Range = Range(i);
                                        end
                                    end
                                    if spwRight(i)>0.2
                                        if Range(i)<P3Range
                                            P3ID = uint8(i);
                                            P3Range = Range(i);
                                        end
                                    end
                                end
                            end
                        end
                    end
                end
            else
                temp = interpolate(single(5),single(10),single(30),single(20),vRef);
                
                if TargetReplacedCnt>4   % no Target lost  Or  After Target 4  cnt!
                    if ((Range(k)<=(TarLimS0Dx+temp))&&(MoveSts(k)==1))||((Range(k)<=(TarLimDx+temp))&&((MoveSts(k)==2)||(MoveSts(k)==3)))
                        if (plaus(k)>=0.2)||((wCutIn(k)>0.6)&&(spw(k)>=0.4))||(spw(k)>0.6)
                            if Range(k)<P0Range
                                P0ID = uint8(k);
                                P0Range = Range(k);
                            end
                        else
                            if spwLeft(k)>0.2
                                if Range(k)<P2Range
                                    P2ID = uint8(k);
                                    P2Range = Range(k);
                                end
                            end
                            if spwLeft(k)>0.2
                                if Range(k)<P3Range
                                    P3ID = uint8(k);
                                    P3Range = Range(k);
                                end
                            end
                        end
                    end
                else  % After lost Target  Replaced  1\2\3 Cnt ！
                    if (Range(k)<(TarLimDx+temp))
                        if (spw(k)>=0.8)||((wCutIn(k)>0.7)&&(spw(k)>=0.4))
                            if Range(k)<P0Range
                                P0ID = uint8(k);
                                P0Range = Range(k);
                            end
                        else
                            if spwLeft(k)>0.2
                                if Range(k)<P2Range
                                    P2ID = uint8(k);
                                    P2Range = Range(k);
                                end
                            end
                            if spwLeft(k)>0.2
                                if Range(k)<P3Range
                                    P3ID = uint8(k);
                                    P3Range = Range(k);
                                end
                            end
                        end
                    end
                end %  After lost Target Replaced  //end 
                for i=1:15
                    if (i~=k)&&(Valid(i)==1)&&...
                            (((vRef<=15.83)&&((MoveSts(i)==1)||(MoveSts(i)==2)||(MoveSts(i)==3)))||...
                            ((vRef>15.83)&&((MoveSts(i)==2)||(MoveSts(i)==3))))
                        if (Classfication(i)==1)||(Classfication(i)==2)||(Classfication(i)==3)||(Classfication(i)==9)
                            if ((Range(i)<=TarLimS0Dx)&&(MoveSts(i)==1))||((Range(i)<=TarLimDx)&&((MoveSts(i)==2)||(MoveSts(i)==3)))
                                if (plaus(i)>=0.4)||((wCutIn(i)>0.7)&&(spw(i)>=0.8))||((spw(i)>0.95)&&(Range(i)<1.5*vRef))
                                    if Range(i)<P0Range
                                        P0ID = uint8(i);
                                        P0Range = Range(i);
                                    end
                                else
                                    if spwLeft(i)>0.2
                                        if Range(i)<P2Range
                                            P2ID = uint8(i);
                                            P2Range = Range(i);
                                        end
                                    end
                                    if spwRight(i)>0.2
                                        if Range(i)<P3Range
                                            P3ID = uint8(i);
                                            P3Range = Range(i);
                                        end
                                    end
                                end
                            end
                        end
                    end
                end
            end
        else
            temp = interpolate(single(5),single(10),single(30),single(20),vRef);
            if (ReRange<(TarLimDx+temp))&&(tTargetLost<0.6)
                if (ReDyc<(DycOffset + dyLaneWidth))&&(ReDyc>(-dyLaneWidth - DycOffset))
                   P0ID = k;
                   P0Range = ReRange;
                end
            end
            for i=1:15
                if (Valid(i)==1)&&...
                        (((vRef<=15.83)&&((MoveSts(i)==1)||(MoveSts(i)==2)||(MoveSts(i)==3)))||...
                        ((vRef>15.83)&&((MoveSts(i)==2)||(MoveSts(i)==3))))
                    if (Classfication(i)==1)||(Classfication(i)==2)||(Classfication(i)==3)||(Classfication(i)==9)
                        if ((Range(i)<=TarLimS0Dx)&&(MoveSts(i)==1))||((Range(i)<=TarLimDx)&&((MoveSts(i)==2)||(MoveSts(i)==3)))
                            if (plaus(i)>=0.4)||((wCutIn(i)>0.7)&&(spw(i)>=0.8))||((spw(i)>0.95)&&(Range(i)<1.5*vRef))
                                if Range(i)<P0Range
                                    P0ID = uint8(i);
                                    P0Range = Range(i);
                                end
                            else
                                if spwLeft(i)>0.2
                                    if Range(i)<P2Range
                                        P2ID = uint8(i);
                                        P2Range = Range(i);
                                    end
                                end
                                if spwRight(i)>0.2
                                    if Range(i)<P3Range
                                        P3ID = uint8(i);
                                        P3Range = Range(i);
                                    end
                                end
                            end
                        end
                    end
                end
            end           
        end
    end
end

if (P0ID>0)&&(P0ID<100)
    TargetExist = true;
    P0Range = Range(P0ID);
    P0Vr = Vr(P0ID);
    P0ArG = ArG(P0ID);
    P0Dx = Dx(P0ID);
    P0Dy = Dy(P0ID);
    if wCutIn(P0ID)>0.6
       TargetCutIn_b = true;
    end
    P0Dyc = Dyc(P0ID);
    P0Vyc = Vyc(P0ID);
else
    if P0ID>100
        TargetExist = true;
        P0Range = ReRange;
        P0Vr = ReVx;
        P0ArG = ReArG;
        P0Dx = ReDx;
        P0Dy = ReDy;
        TargetCutIn_b = ReCutIn_b;
        P0Dyc = ReDyc;
        P0Vyc = ReVyc;
    end
end
if P2ID>0
    P2Range = Range(P2ID);
    P2Vr = Vr(P2ID);
    P2ArG = ArG(P2ID);
    P2Dx = Dx(P2ID);
    P2Dy = Dy(P2ID);
end
if P3ID>0
    P3Range = Range(P3ID);
    P3Vr = Vr(P3ID);
    P3ArG = ArG(P3ID);
    P3Dx = Dx(P3ID);
    P3Dy = Dy(P3ID);
end
end
